simulink model "Gep_Lab3_A4"  (R2020b)
settings: Solver=VariableStepAuto  StartTime=0.0  StopTime=0.2  MaxStep=10e-6  RelTol=1e-6
undefined symbols (not defined in the file): alpha, plecs
settings Model: Creator=barac  LastModifiedBy=barac

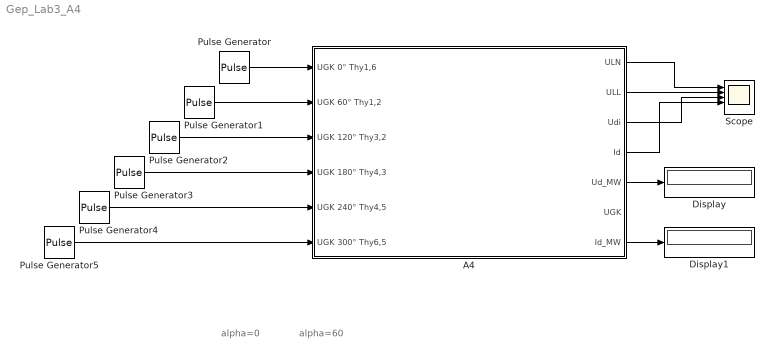
== system Gep_Lab3_A4 ==
  note: alpha=0
  note: alpha=60
  A4 : Subsystem  LoadFcn=plecs('sl', 200);  InitFcn=plecs('sl', 214);  StartFcn=plecs('sl', 208);  StopFcn=plecs('sl', 209);  mask(PlecsCircuit){PLECSData=<binary blob, 5384 chars, not shown>}
      mask prompts: PLECSData "PLECS Data (Do not delete or modify!)"
      mask init:
      | % PLACE CUSTOM INITIALIZATIONS ABOVE
      | % DO NOT REMOVE
      | plecs('sl', 215);
      | % DO NOT REMOVE
      settings: CopyFcn=plecs('sl', 203);  DeleteFcn=plecs('sl', 205);  UndoDeleteFcn=plecs('sl', 206);  PreSaveFcn=plecs('sl', 211);  PostSaveFcn=plecs('sl', 201);  NameChangeFcn=plecs('sl', 210);  DestroyFcn=plecs('sl', 207);  PreCopyFcn=plecs('sl', 216);  OpenFcn=plecs('sl', 202);  ErrorFcn=plerrorfcn
      mask Help: web(['file:///' fullfile(plecsdoc, 'creatingacircuit.html')])
      mask Display: disp('PLECS\nCircuit')
  Display : Display
  Display1 : Display
  Pulse Generator : DiscretePulseGenerator  PulseType=Time based  Period=1/50  PulseWidth=5  PhaseDelay=((1/50)/180)*(30+alpha)
  Pulse Generator1 : DiscretePulseGenerator  PulseType=Time based  Period=0.02  PulseWidth=5  PhaseDelay=((1/50)/360)*(alpha+60+30)
  Pulse Generator2 : DiscretePulseGenerator  PulseType=Time based  Period=0.02  PulseWidth=5  PhaseDelay=((1/50)/360)*(alpha+120+30)
  Pulse Generator3 : DiscretePulseGenerator  PulseType=Time based  Period=0.02  PulseWidth=5  PhaseDelay=((1/50)/360)*(alpha+180+30)
  Pulse Generator4 : DiscretePulseGenerator  PulseType=Time based  Period=0.02  PulseWidth=5  PhaseDelay=((1/50)/360)*(alpha+240+30)
  Pulse Generator5 : DiscretePulseGenerator  PulseType=Time based  Period=0.02  PulseWidth=5  PhaseDelay=((1/50)/360)*(alpha+300+30)
  Scope : Scope  NumInputPorts=5
  wires:
  Pulse Generator/1 -> A4/1(UGK 0° Thy1,6)
  Pulse Generator1/1 -> A4/2(UGK 60° Thy1,2)
  Pulse Generator2/1 -> A4/3(UGK 120° Thy3,2)
  Pulse Generator3/1 -> A4/4(UGK 180° Thy4,3)
  Pulse Generator4/1 -> A4/5(UGK 240° Thy4,5)
  Pulse Generator5/1 -> A4/6(UGK 300° Thy6,5)
  A4/1(ULN) -> Scope/1
  A4/2(ULL) -> Scope/2
  A4/3(Udi) -> Scope/3
  A4/4(Id) -> Scope/4
  A4/5(Ud_MW) -> Display/1
  A4/7(Id_MW) -> Display1/1

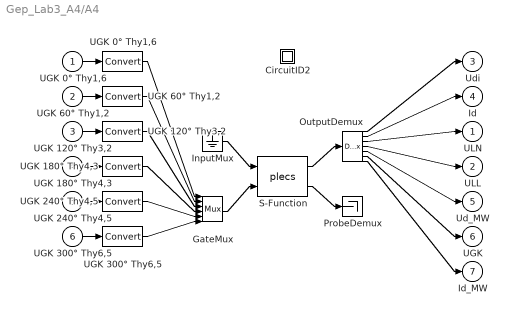
== system Gep_Lab3_A4/A4 ==
  UGK 0° Thy1,6 : Inport  PortDimensions=1
  UGK 60° Thy1,2 : Inport  Port=2  PortDimensions=1
  UGK 120° Thy3,2 : Inport  Port=3  PortDimensions=1
  UGK 180° Thy4,3 : Inport  Port=4  PortDimensions=1
  UGK 240° Thy4,5 : Inport  Port=5  PortDimensions=1
  UGK 300° Thy6,5 : Inport  Port=6  PortDimensions=1
  " CircuitID2 " : Subsystem
  " GateMux " : Mux  Inputs=[ 1 1 1 1 1 1 ]
  " InputMux " : Ground
  " OutputDemux " : Demux  Outputs=[ 1 1 3 3 1 6 1 ]
  " ProbeDemux " : Terminator
  " S-Function " : S-Function  FunctionName=plecs  SFunctionDeploymentMode=off  EnableBusSupport=off
  " UGK 0° Thy1,6 " : DataTypeConversion  SaturateOnIntegerOverflow=on  RndMeth=Zero
  " UGK 120° Thy3,2 " : DataTypeConversion  SaturateOnIntegerOverflow=on  RndMeth=Zero
  " UGK 180° Thy4,3 " : DataTypeConversion  SaturateOnIntegerOverflow=on  RndMeth=Zero
  " UGK 240° Thy4,5 " : DataTypeConversion  SaturateOnIntegerOverflow=on  RndMeth=Zero
  " UGK 300° Thy6,5 " : DataTypeConversion  SaturateOnIntegerOverflow=on  RndMeth=Zero
  " UGK 60° Thy1,2 " : DataTypeConversion  SaturateOnIntegerOverflow=on  RndMeth=Zero
  ULN : Outport  PortDimensions=3
  ULL : Outport  Port=2  PortDimensions=3
  Udi : Outport  Port=3  PortDimensions=1
  Id : Outport  Port=4  PortDimensions=1
  Ud_MW : Outport  Port=5  PortDimensions=1
  UGK : Outport  Port=6  PortDimensions=6
  Id_MW : Outport  Port=7  PortDimensions=1
  wires:
  " InputMux "/1 -> " S-Function "/1
  " GateMux "/1 -> " S-Function "/2
  " S-Function "/1 -> " OutputDemux "/1
  " S-Function "/2 -> " ProbeDemux "/1
  UGK 0° Thy1,6/1 -> " UGK 0° Thy1,6 "/1
  " UGK 0° Thy1,6 "/1 -> " GateMux "/1
  UGK 60° Thy1,2/1 -> " UGK 60° Thy1,2 "/1
  " UGK 60° Thy1,2 "/1 -> " GateMux "/2
  UGK 120° Thy3,2/1 -> " UGK 120° Thy3,2 "/1
  " UGK 120° Thy3,2 "/1 -> " GateMux "/3
  UGK 180° Thy4,3/1 -> " UGK 180° Thy4,3 "/1
  " UGK 180° Thy4,3 "/1 -> " GateMux "/4
  UGK 240° Thy4,5/1 -> " UGK 240° Thy4,5 "/1
  " UGK 240° Thy4,5 "/1 -> " GateMux "/5
  UGK 300° Thy6,5/1 -> " UGK 300° Thy6,5 "/1
  " UGK 300° Thy6,5 "/1 -> " GateMux "/6
  " OutputDemux "/1 -> Udi/1
  " OutputDemux "/2 -> Id/1
  " OutputDemux "/3 -> ULN/1
  " OutputDemux "/4 -> ULL/1
  " OutputDemux "/5 -> Ud_MW/1
  " OutputDemux "/6 -> UGK/1
  " OutputDemux "/7 -> Id_MW/1

== system Gep_Lab3_A4/A4/ CircuitID2  ==
